simulink model "c28x_i2c_sensor"  (R2021b)
settings: Solver=FixedStepDiscrete  StartTime=0.0  StopTime=Inf  FixedStep=Auto  RelTol=1e-3  EnableMultiTasking=on
libraries: simulink x8, c280xlib x7, demo_controls x1
settings Model: SimulationMode=external  ExtModeTrigDuration=8  Creator=The MathWorks, Inc.  LastModifiedBy=The MathWorks, Inc.
settings SolverCC: AlgebraicLoopSolver=TrustRegion
settings DataIOCC: LimitDataPoints=on  SaveFormat=Array  SaveOutput=off  SaveTime=off  ReturnWorkspaceOutputs=off
settings OptimizationCC: BlockReduction=off  ConditionallyExecuteInputs=off  DefaultUnderspecifiedDataType=single  OptimizeBlockIOStorage=off  BufferReuse=off  GlobalBufferReuse=off  ExpressionFolding=off  ExpressionDepthLimit=2147483647  LocalBlockOutputs=off  InitFltsAndDblsToZero=on  LifeSpan=Inf  MaxStackSize=512  EfficientTunableParamExpr=on
settings DebuggingCC: UnderspecifiedInitializationDetection=Classic  MergeDetectMultiDrivingBlocksExec=none  SolverPrmCheckMsg=warning  InheritedTsInSrcMsg=none  FcnCallInpInsideContextMsg=warning  AllowSymbolicDim=off  StateNameClashWarn=warning  SFUnexpectedBacktrackingDiag=warning  SFNoUnconditionalDefaultTransitionDiag=warning  SFExecutionAtInitializationDiag=none  SFMachineParentedDataDiag=warning  ArithmeticOperatorsInVariantConditions=warning
settings HardwareCC: ProdBitPerChar=16  ProdBitPerInt=16  ProdBitPerPointer=32  ProdBitPerSizeT=32  ProdBitPerPtrDiffT=32  ProdLargestAtomicInteger=Integer  ProdLargestAtomicFloat=None  ProdWordSize=16  ProdLongLongMode=on  ProdHWDeviceType=Texas Instruments->C2000  TargetBitPerChar=16  TargetBitPerInt=16  TargetBitPerPointer=16  TargetIntDivRoundTo=Zero  TargetEndianess=LittleEndian  TargetWordSize=16  TargetHWDeviceType=TI C2000
settings ModelReferenceCC: ModelReferenceNumInstancesAllowed=Single  PropagateSignalLabelsOutOfModel=off
settings SFSimCC: SimUseLocalCustomCode=off  SimParseCustomCode=off  CustomCodeUndefinedFunction=UseInterfaceOnly
settings RTWCC: Description=Embedded Coder  SystemTargetFile=ert.tlc  HardwareBoard=TI Delfino F2837xS  TemplateMakefile=ert_default_tmf  RTWUseLocalCustomCode=off  Toolchain=Texas Instruments Code Composer Studio (C2000)
settings CodeAppCC: IgnoreCustomStorageClasses=off  CustomSymbolStrType=$N$R$M  StateflowObjectComments=on  InternalIdentifier=Classic
settings ERTTargetCC: CodeReplacementLibrary=TI C28x  MultiwordLength=2048  ExtModeTransport=4  ExtModeStaticAlloc=on  ExtModeStaticAllocSize=10000  ExtModeMexFile=ext_xcp  ExtModeIntrfLevel=Level2 - Open  ConvertIfToSwitch=off  SuppressUnreachableDefaultCases=off
settings ConfigComp: CovMetricSettings=dw  CovSaveCumulativeToWorkspaceVar=on  CovSaveSingleToWorkspaceVar=on  CovExternalEMLEnable=off  CovSFcnEnable=off

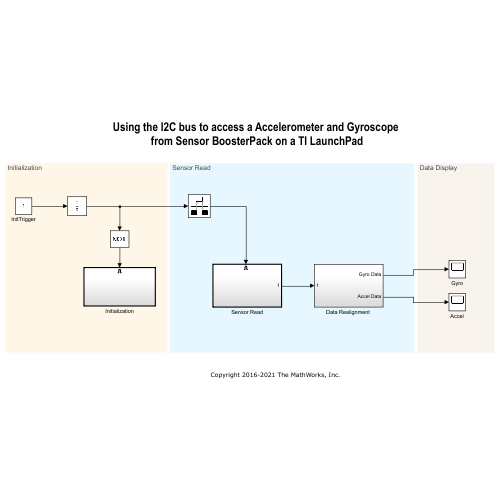
[thumbnail: Simulink's stored preview of the top-level diagram]
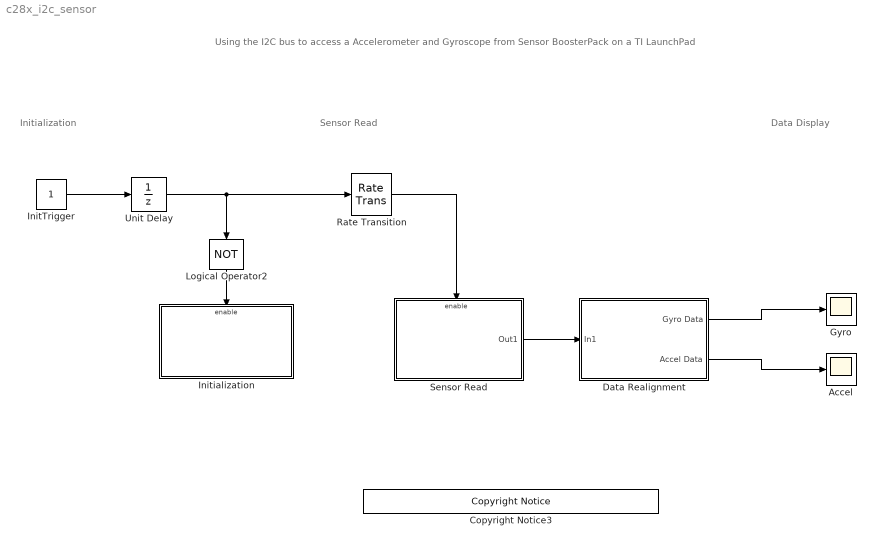
== system c28x_i2c_sensor ==
  note: Using the I2C bus to access a Accelerometer and Gyroscope
      | from Sensor BoosterPack on a TI LaunchPad
  note: Initialization
  note: Data Display
  note: Sensor Read
  Accel : Scope
  Copyright Notice3 : demo_controls/Copyright Notice  year=2016  prod=tic2000
      settings: SourceProductBaseCode=ME
  "Data Realignment " : Subsystem
  Gyro : Scope
  InitTrigger : Constant  Priority=10  OutDataTypeStr=uint16  SampleTime=15e-3
  Initialization : Subsystem
  Logical Operator2 : Logic  Operator=NOT  AllPortsSameDT=off  OutDataTypeStr=boolean
  Rate Transition : RateTransition  OutPortSampleTime=1e-3
  Sensor Read : Subsystem  Priority=10  TreatAsAtomicUnit=on
  Unit Delay : UnitDelay  SampleTime=-1  HasFrameUpgradeWarning=on
  wires:
  Sensor Read/1(Out1) -> "Data Realignment "/1(In1)
  Unit Delay/1 -> Rate Transition/1, Logical Operator2/1
  "Data Realignment "/1(Gyro Data) -> Gyro/1
  "Data Realignment "/2(Accel Data) -> Accel/1
  Logical Operator2/1 -> Initialization/Enable
  Rate Transition/1 -> Sensor Read/Enable
  InitTrigger/1 -> Unit Delay/1

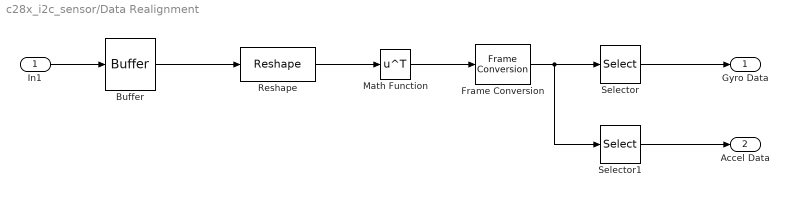
== system c28x_i2c_sensor/Data Realignment  ==
  In1 : Inport
  Buffer : Buffer  N=30*6
  Frame Conversion : FrameConversion
  Math Function : Math  Operator=transpose  SignedPower=on  SaturateOnIntegerOverflow=on
  Reshape : Reshape  OutputDimensionality=Customize  OutputDimensions=[6,30]
  Selector : Selector  NumberOfDimensions=2  InputPortWidth=3  IndexOptions=Index vector (dialog),Starting index (dialog)  Indices=1:30,1  OutputSizes=1,3
  Selector1 : Selector  NumberOfDimensions=2  InputPortWidth=3  IndexOptions=Index vector (dialog),Starting index (dialog)  Indices=1:30,4  OutputSizes=1,3
  Gyro Data : Outport  VectorParamsAs1DForOutWhenUnconnected=off
  Accel Data : Outport  Port=2  VectorParamsAs1DForOutWhenUnconnected=off
  wires:
  In1/1 -> Buffer/1
  Reshape/1 -> Math Function/1
  Buffer/1 -> Reshape/1
  Frame Conversion/1 -> Selector1/1, Selector/1
  Math Function/1 -> Frame Conversion/1
  Selector/1 -> Gyro Data/1
  Selector1/1 -> Accel Data/1

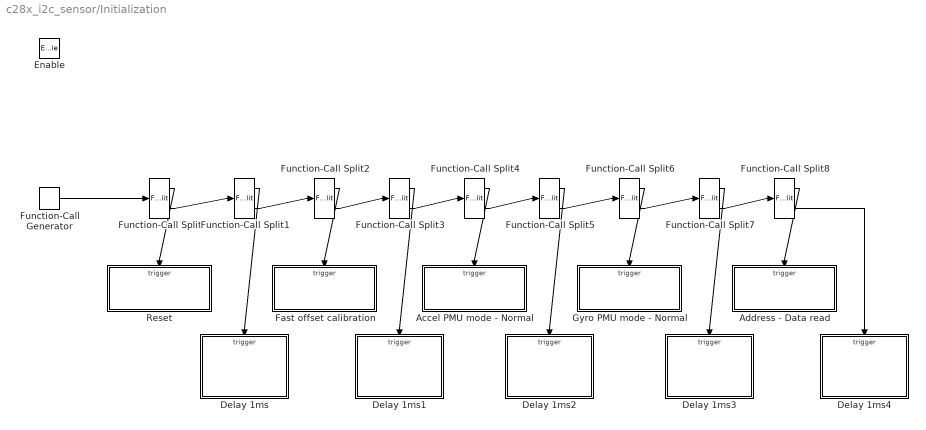
== system c28x_i2c_sensor/Initialization ==
  Enable : EnablePort
  Accel PMU mode - Normal : Subsystem  TreatAsAtomicUnit=on
  Address - Data read : Subsystem  TreatAsAtomicUnit=on
  Delay 1ms : Subsystem  TreatAsAtomicUnit=on
  Delay 1ms1 : Subsystem  TreatAsAtomicUnit=on
  Delay 1ms2 : Subsystem  TreatAsAtomicUnit=on
  Delay 1ms3 : Subsystem  TreatAsAtomicUnit=on
  Delay 1ms4 : Subsystem  TreatAsAtomicUnit=on
  Fast offset calibration : Subsystem  TreatAsAtomicUnit=on
  Function-Call Generator : simulink/Ports & Subsystems/Function-Call Generator  sample_time=-1  numberOfIterations=1  DisallowWideOutput=off
  Function-Call Split{,1..8} (9 alike) : FunctionCallSplit  NumOutputPorts=2
  Gyro PMU mode - Normal : Subsystem  TreatAsAtomicUnit=on
  Reset : Subsystem  TreatAsAtomicUnit=on
  wires:
  Function-Call Split4/1 -> Accel PMU mode - Normal/Trigger
  Function-Call Split3/2 -> Function-Call Split4/1
  Function-Call Split1/1 -> Delay 1ms/Trigger
  Function-Call Split2/1 -> Fast offset calibration/Trigger
  Function-Call Split5/2 -> Function-Call Split6/1
  Function-Call Split/2 -> Function-Call Split1/1
  Function-Call Split1/2 -> Function-Call Split2/1
  Function-Call Split8/1 -> Address - Data read/Trigger
  Function-Call Split6/2 -> Function-Call Split7/1
  Function-Call Split4/2 -> Function-Call Split5/1
  Function-Call Generator/1 -> Function-Call Split/1
  Function-Call Split7/1 -> Delay 1ms3/Trigger
  Function-Call Split7/2 -> Function-Call Split8/1
  Function-Call Split5/1 -> Delay 1ms2/Trigger
  Function-Call Split/1 -> Reset/Trigger
  Function-Call Split3/1 -> Delay 1ms1/Trigger
  Function-Call Split8/2 -> Delay 1ms4/Trigger
  Function-Call Split6/1 -> Gyro PMU mode - Normal/Trigger
  Function-Call Split2/2 -> Function-Call Split3/1

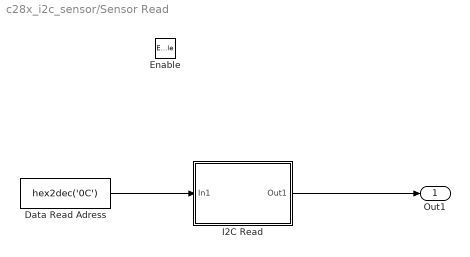
== system c28x_i2c_sensor/Sensor Read ==
  Enable : EnablePort
  Data Read Adress : Constant  Priority=10  Value=hex2dec('0C')  OutDataTypeStr=uint8  SampleTime=-1
  I2C Read : Subsystem
  Out1 : Outport  InitialOutput=[0 0 0 0 0 0]  VectorParamsAs1DForOutWhenUnconnected=off
  wires:
  Data Read Adress/1 -> I2C Read/1(In1)
  I2C Read/1(Out1) -> Out1/1

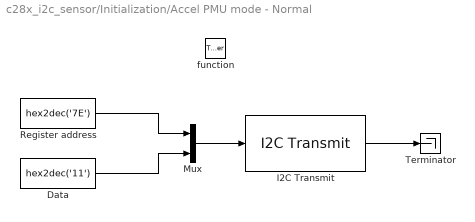
== system c28x_i2c_sensor/Initialization/Accel PMU mode - Normal ==
  function : TriggerPort  TriggerType=function-call  VariantControl=Variant
  Data : Constant  Value=hex2dec('11')  OutDataTypeStr=uint8  SampleTime=-1
  I2C Transmit : c280xlib/I2C Transmit  selectModule=I2C_A  addrFormat=7-Bit addressing  saSource=Specify via dialog  SAR=105  bitCount=8  STP=on  RM=off  STR=on
      settings: SourceProductBaseCode=TIC2000
  Mux : Mux  Inputs=2
  Register address : Constant  Value=hex2dec('7E')  OutDataTypeStr=uint8  SampleTime=-1
  Terminator : Terminator
  wires:
  Register address/1 -> Mux/1
  Data/1 -> Mux/2
  I2C Transmit/1 -> Terminator/1
  Mux/1 -> I2C Transmit/1

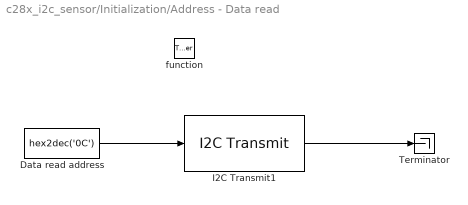
== system c28x_i2c_sensor/Initialization/Address - Data read ==
  function : TriggerPort  TriggerType=function-call  VariantControl=Variant
  Data read address : Constant  Value=hex2dec('0C')  OutDataTypeStr=uint8  SampleTime=-1
  I2C Transmit1 : c280xlib/I2C Transmit  selectModule=I2C_A  addrFormat=7-Bit addressing  saSource=Specify via dialog  SAR=105  bitCount=8  STP=off  RM=off  STR=on
      settings: SourceProductBaseCode=TIC2000
  Terminator : Terminator
  wires:
  Data read address/1 -> I2C Transmit1/1
  I2C Transmit1/1 -> Terminator/1

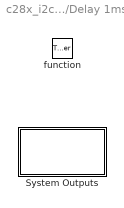
== system c28x_i2c_sensor/Initialization/Delay 1ms ==
  function : TriggerPort  TriggerType=function-call  VariantControl=Variant
  System Outputs : Subsystem  mask(System Outputs){ShowInLibBrowser=0}
      mask prompts: ShowInLibBrowser "Simulink:masks:CustCodeMaskParam1_MP"
      settings: CopyFcn=cccopyfcn(gcb)  OpenFcn=ccopenfcn('System Outputs Function')
      mask Help: eval('feval(''rtwprivate'',''rtwhelpview'',''rtw_sys_outputs_block'')');
      mask Display: disp('System\nOutputs');

== system c28x_i2c_sensor/Initialization/Delay 1ms1 ==
  function : TriggerPort  TriggerType=function-call  VariantControl=Variant
  System Outputs : Subsystem  mask(System Outputs){ShowInLibBrowser=0}
      mask prompts: ShowInLibBrowser "Simulink:masks:CustCodeMaskParam1_MP"
      settings: CopyFcn=cccopyfcn(gcb)  OpenFcn=ccopenfcn('System Outputs Function')
      mask Help: eval('feval(''rtwprivate'',''rtwhelpview'',''rtw_sys_outputs_block'')');
      mask Display: disp('System\nOutputs');

== system c28x_i2c_sensor/Initialization/Delay 1ms2 ==
  function : TriggerPort  TriggerType=function-call  VariantControl=Variant
  System Outputs : Subsystem  mask(System Outputs){ShowInLibBrowser=0}
      mask prompts: ShowInLibBrowser "Simulink:masks:CustCodeMaskParam1_MP"
      settings: CopyFcn=cccopyfcn(gcb)  OpenFcn=ccopenfcn('System Outputs Function')
      mask Help: eval('feval(''rtwprivate'',''rtwhelpview'',''rtw_sys_outputs_block'')');
      mask Display: disp('System\nOutputs');

== system c28x_i2c_sensor/Initialization/Delay 1ms3 ==
  function : TriggerPort  TriggerType=function-call  VariantControl=Variant
  System Outputs : Subsystem  mask(System Outputs){ShowInLibBrowser=0}
      mask prompts: ShowInLibBrowser "Simulink:masks:CustCodeMaskParam1_MP"
      settings: CopyFcn=cccopyfcn(gcb)  OpenFcn=ccopenfcn('System Outputs Function')
      mask Help: eval('feval(''rtwprivate'',''rtwhelpview'',''rtw_sys_outputs_block'')');
      mask Display: disp('System\nOutputs');

== system c28x_i2c_sensor/Initialization/Delay 1ms4 ==
  function : TriggerPort  TriggerType=function-call  VariantControl=Variant
  System Outputs : Subsystem  mask(System Outputs){ShowInLibBrowser=0}
      mask prompts: ShowInLibBrowser "Simulink:masks:CustCodeMaskParam1_MP"
      settings: CopyFcn=cccopyfcn(gcb)  OpenFcn=ccopenfcn('System Outputs Function')
      mask Help: eval('feval(''rtwprivate'',''rtwhelpview'',''rtw_sys_outputs_block'')');
      mask Display: disp('System\nOutputs');

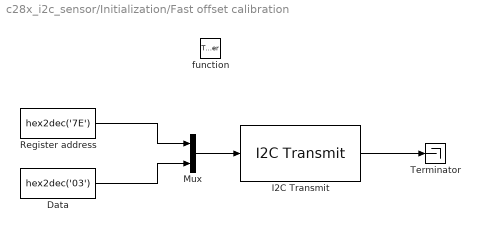
== system c28x_i2c_sensor/Initialization/Fast offset calibration ==
  function : TriggerPort  TriggerType=function-call  VariantControl=Variant
  Data : Constant  Value=hex2dec('03')  OutDataTypeStr=uint8  SampleTime=-1
  I2C Transmit : c280xlib/I2C Transmit  selectModule=I2C_A  addrFormat=7-Bit addressing  saSource=Specify via dialog  SAR=105  bitCount=8  STP=on  RM=off  STR=on
      settings: SourceProductBaseCode=TIC2000
  Mux : Mux  Inputs=2
  Register address : Constant  Value=hex2dec('7E')  OutDataTypeStr=uint8  SampleTime=-1
  Terminator : Terminator
  wires:
  Data/1 -> Mux/2
  I2C Transmit/1 -> Terminator/1
  Mux/1 -> I2C Transmit/1
  Register address/1 -> Mux/1

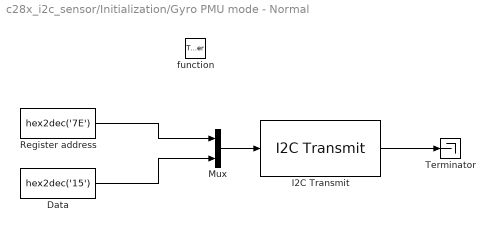
== system c28x_i2c_sensor/Initialization/Gyro PMU mode - Normal ==
  function : TriggerPort  TriggerType=function-call  VariantControl=Variant
  Data : Constant  Value=hex2dec('15')  OutDataTypeStr=uint8  SampleTime=-1
  I2C Transmit : c280xlib/I2C Transmit  selectModule=I2C_A  addrFormat=7-Bit addressing  saSource=Specify via dialog  SAR=105  bitCount=8  STP=on  RM=off  STR=on
      settings: SourceProductBaseCode=TIC2000
  Mux : Mux  Inputs=2
  Register address : Constant  Value=hex2dec('7E')  OutDataTypeStr=uint8  SampleTime=-1
  Terminator : Terminator
  wires:
  I2C Transmit/1 -> Terminator/1
  Mux/1 -> I2C Transmit/1
  Register address/1 -> Mux/1
  Data/1 -> Mux/2

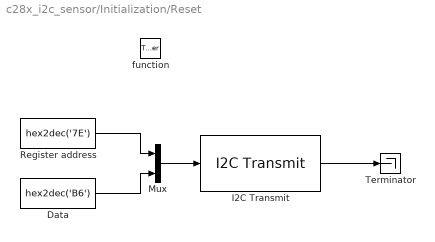
== system c28x_i2c_sensor/Initialization/Reset ==
  function : TriggerPort  TriggerType=function-call  VariantControl=Variant
  Data : Constant  Value=hex2dec('B6')  OutDataTypeStr=uint8  SampleTime=-1
  I2C Transmit : c280xlib/I2C Transmit  selectModule=I2C_A  addrFormat=7-Bit addressing  saSource=Specify via dialog  SAR=105  bitCount=8  STP=on  RM=off  STR=on
      settings: SourceProductBaseCode=TIC2000
  Mux : Mux  Inputs=2
  Register address : Constant  Value=hex2dec('7E')  OutDataTypeStr=uint8  SampleTime=-1
  Terminator : Terminator
  wires:
  Data/1 -> Mux/2
  Register address/1 -> Mux/1
  I2C Transmit/1 -> Terminator/1
  Mux/1 -> I2C Transmit/1

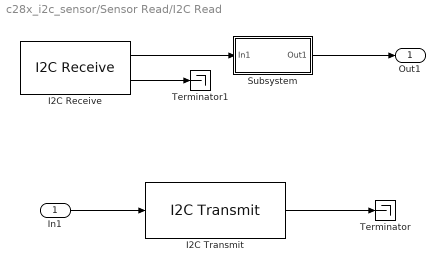
== system c28x_i2c_sensor/Sensor Read/I2C Read ==
  In1 : Inport
  I2C Receive : c280xlib/I2C Receive  Priority=10  selectModule=I2C_A  addrFormat=7-Bit addressing  saSource=Specify via dialog  SAR=105  bitCount=8  dataLength=12  initValue=0  NACK=off  STP=on  STR=on  sampleTime=-1  dataType=uint8
      settings: SourceProductBaseCode=TIC2000
  I2C Transmit : c280xlib/I2C Transmit  Priority=20  selectModule=I2C_A  addrFormat=7-Bit addressing  saSource=Specify via dialog  SAR=105  bitCount=8  STP=off  RM=off  STR=on
      settings: SourceProductBaseCode=TIC2000
  Subsystem : Subsystem
  Terminator : Terminator
  Terminator1 : Terminator
  Out1 : Outport  VectorParamsAs1DForOutWhenUnconnected=off
  wires:
  In1/1 -> I2C Transmit/1
  I2C Receive/1 -> Subsystem/1(In1)
  I2C Receive/2 -> Terminator1/1
  Subsystem/1(Out1) -> Out1/1
  I2C Transmit/1 -> Terminator/1

== system c28x_i2c_sensor/Initialization/Delay 1ms/System Outputs ==

== system c28x_i2c_sensor/Initialization/Delay 1ms1/System Outputs ==

== system c28x_i2c_sensor/Initialization/Delay 1ms2/System Outputs ==

== system c28x_i2c_sensor/Initialization/Delay 1ms3/System Outputs ==

== system c28x_i2c_sensor/Initialization/Delay 1ms4/System Outputs ==

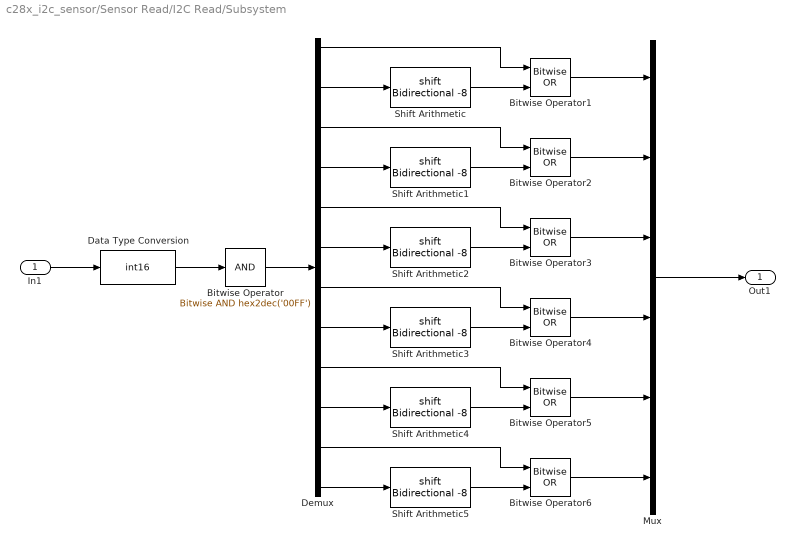
== system c28x_i2c_sensor/Sensor Read/I2C Read/Subsystem ==
  In1 : Inport
  Bitwise Operator : simulink/Logic and Bit Operations/Bitwise Operator  logicop=AND  UseBitMask=on  BitMask=hex2dec('00FF')  BitMaskRealWorld=Stored Integer
  Bitwise Operator{1..6} (6 alike) : simulink/Logic and Bit Operations/Bitwise Operator  logicop=OR  UseBitMask=off  NumInputPorts=2  BitMask=bin2dec('11011001')  BitMaskRealWorld=Stored Integer
  Data Type Conversion : DataTypeConversion  OutDataTypeStr=int16  ConvertRealWorld=Stored Integer (SI)
  Demux : Demux  Outputs=12
  Mux : Mux  Inputs=6
  Shift Arithmetic{,1..5} (6 alike) : ArithShift  BitShiftNumber=-8
  Out1 : Outport  VectorParamsAs1DForOutWhenUnconnected=off
  wires:
  In1/1 -> Data Type Conversion/1
  Data Type Conversion/1 -> Bitwise Operator/1
  Mux/1 -> Out1/1
  Bitwise Operator/1 -> Demux/1
  Bitwise Operator4/1 -> Mux/4
  Bitwise Operator5/1 -> Mux/5
  Bitwise Operator3/1 -> Mux/3
  Bitwise Operator6/1 -> Mux/6
  Bitwise Operator1/1 -> Mux/1
  Bitwise Operator2/1 -> Mux/2
  Demux/1 -> Bitwise Operator1/1
  Demux/2 -> Shift Arithmetic/1
  Shift Arithmetic/1 -> Bitwise Operator1/2
  Demux/3 -> Bitwise Operator2/1
  Demux/4 -> Shift Arithmetic1/1
  Shift Arithmetic1/1 -> Bitwise Operator2/2
  Demux/5 -> Bitwise Operator3/1
  Shift Arithmetic2/1 -> Bitwise Operator3/2
  Demux/6 -> Shift Arithmetic2/1
  Demux/7 -> Bitwise Operator4/1
  Demux/8 -> Shift Arithmetic3/1
  Demux/9 -> Bitwise Operator5/1
  Demux/10 -> Shift Arithmetic4/1
  Demux/11 -> Bitwise Operator6/1
  Demux/12 -> Shift Arithmetic5/1
  Shift Arithmetic3/1 -> Bitwise Operator4/2
  Shift Arithmetic4/1 -> Bitwise Operator5/2
  Shift Arithmetic5/1 -> Bitwise Operator6/2
